simulink model "mymodel1"  (R2018a)
settings: Solver=VariableStepAuto  StartTime=0.0  StopTime=10.0  RelTol=1e-3
libraries: xbsIndex_r4 x12453, casper_library_misc x30, casper_library_delays x14, xps_library x2
(part 21 of 108)

== system mymodel1/pfb_fir_generic/pfb_fir_taps/bus_mult ==
  a : Inport
  b : Inport  Port=2
  a*b_bussify : Subsystem  AncestorBlock=casper_library_flow_control/bus_create  mask(bus_create){inputNum=96}
      mask prompts: inputNum "Number of inputs:"
      mask init:
      | bus_create_init(gcb,...
      |     'inputNum', inputNum);
  a_debus : Subsystem  AncestorBlock=casper_library_flow_control/bus_expand  mask(bus_expand){mode=divisions of arbitrary size, outputNum=1, outputWidth=[16 16 16 16 16 16 16 16 16 16 16 16 16 16 16 16 16 16 16 16 16 16 16 16 16 16 16 16 16 16 16 16 16 16 16 16 16 16 16 16 16 16 16 16 16 16 16 16 16 16 16 16 16 16 16 16 16 16 16 16 16 16 16 16 16 16 16 16 16 16 16 16 16 16 16 16 16 16 16 16 16 16 16 16 16 16 16 16 16 16 16 16 16 16 16 16], outputBinaryPt=[15 15 15 15 15 15 15 15 15 15 15 15 15 15 15 15 15 15 15 15 15 15 15 15 15 15 15 15 15 15 15 15 15 15 15 15 15 15 15 15 15 15 15 15 15 15 15 15 15 15 15 15 15 15 15 15 15 15 15 15 15 15 15 15 15 15 15 15 15 15 15 15 15 15 15 15 15 15 15 15 15 15 15 15 15 15 15 15 15 15 15 15 15 15 15 15], outputArithmeticType=[1 1 1 1 1 1 1 1 1 1 1 1 1 1 1 1 1 1 1 1 1 1 1 1 1 1 1 1 1 1 1 1 1 1 1 1 1 1 1 1 1 1 1 1 1 1 1 1 1 1 1 1 1 1 1 1 1 1 1 1 1 1 1 1 1 1 1 1 1 1 1 1 1 1 1 1 1 1 1 1 1 1 1 1 1 1 1 1 1 1 1 1 1 1 1 1], show_format=on, outputToWorkspace=off, variablePrefix=, outputToModelAsWell=on}
      mask prompts: outputNum "Number of outputs:"; outputWidth "Output width [msb ... lsb]:"; outputBinaryPt "Output binary point position [msb ... lsb]:"; outputArithmeticType "Output arithmetic type (ufix=0, fix=1, bool=2) [msb ... lsb]:"; show_format "Print format string?"; outputToWorkspace "Output to workspace?"; variablePrefix "Variable name prefix:"; outputToModelAsWell "Output to model as well?"
      mask help:
      | Expands a 'bus' made using a bus_create or Xilinx
      | concat block.
      | The input will be divided into the specified number
      | of outputs with the specified arithmetic types.
      | Divisions are made from most significant bit.
      mask init: same as mymodel1/bit_sel_xx0/bus_expand1
      settings: AttributesFormatString=96 outputs: f16.15,f16.15,f16.15,f16.15,f16.15,f16.15,f16.15,f16.15,f16.15,f16.15,f16.15,f16.15,f16.15,f16.15,f16.15,f16.15,f16.15,f16.15,f16.15,f16.15,f16.15,f16.15,f16.15,f16.15,f16.15,f16.15,f16.15,f16.15,f16.15,f16.15,f16.15,f16.15,f16.15,f16.15,f16.15,f16.15,f16.15,f16.15,f16.15,f16.15,f16.15,f16.15,f16.15,f16.15,f16.15,f16.15,f16.15,f16.15,f16.15,f16.15,f16.15,f16.15,f16.15,f16.15,f16.15,f16.15,f16.15,f16.15,f16.15,f16.15,f16.15,f16.15,f16.15,f16.15,f16.15,f16.15,f16.15,f16.15,f16.15,f16.15,f16.15,f16.15,f16.15,f16.15,f16.15,f16.15,f16.15,f16.15,f16.15,f16.15,f16.15,f16.15,f16.15,f16.15,f16.15,f16.15,f16.15,f16.15,f16.15,f16.15,f16.15,f16.15,f16.15,f16.15,f16.15,f16.15,
      mask TypeOptions mode: divisions of equal size | divisions of arbitrary size
      mask Callback mode: bus_expand_callback();
      mask Callback outputWidth: bus_expand_callback();
      mask Callback outputToWorkspace: bus_expand_callback();
  b_debus : Subsystem  AncestorBlock=casper_library_flow_control/bus_expand  mask(bus_expand){mode=divisions of arbitrary size, outputNum=1, outputWidth=[18 18 18 18 18 18 18 18 18 18 18 18 18 18 18 18 18 18 18 18 18 18 18 18 18 18 18 18 18 18 18 18 18 18 18 18 18 18 18 18 18 18 18 18 18 18 18 18 18 18 18 18 18 18 18 18 18 18 18 18 18 18 18 18 18 18 18 18 18 18 18 18 18 18 18 18 18 18 18 18 18 18 18 18 18 18 18 18 18 18 18 18 18 18 18 18], outputBinaryPt=[17 17 17 17 17 17 17 17 17 17 17 17 17 17 17 17 17 17 17 17 17 17 17 17 17 17 17 17 17 17 17 17 17 17 17 17 17 17 17 17 17 17 17 17 17 17 17 17 17 17 17 17 17 17 17 17 17 17 17 17 17 17 17 17 17 17 17 17 17 17 17 17 17 17 17 17 17 17 17 17 17 17 17 17 17 17 17 17 17 17 17 17 17 17 17 17], outputArithmeticType=[1 1 1 1 1 1 1 1 1 1 1 1 1 1 1 1 1 1 1 1 1 1 1 1 1 1 1 1 1 1 1 1 1 1 1 1 1 1 1 1 1 1 1 1 1 1 1 1 1 1 1 1 1 1 1 1 1 1 1 1 1 1 1 1 1 1 1 1 1 1 1 1 1 1 1 1 1 1 1 1 1 1 1 1 1 1 1 1 1 1 1 1 1 1 1 1], show_format=on, outputToWorkspace=off, variablePrefix=, outputToModelAsWell=on}
      mask prompts: outputNum "Number of outputs:"; outputWidth "Output width [msb ... lsb]:"; outputBinaryPt "Output binary point position [msb ... lsb]:"; outputArithmeticType "Output arithmetic type (ufix=0, fix=1, bool=2) [msb ... lsb]:"; show_format "Print format string?"; outputToWorkspace "Output to workspace?"; variablePrefix "Variable name prefix:"; outputToModelAsWell "Output to model as well?"
      mask help:
      | Expands a 'bus' made using a bus_create or Xilinx
      | concat block.
      | The input will be divided into the specified number
      | of outputs with the specified arithmetic types.
      | Divisions are made from most significant bit.
      mask init: same as mymodel1/bit_sel_xx0/bus_expand1
      settings: AttributesFormatString=96 outputs: f18.17,f18.17,f18.17,f18.17,f18.17,f18.17,f18.17,f18.17,f18.17,f18.17,f18.17,f18.17,f18.17,f18.17,f18.17,f18.17,f18.17,f18.17,f18.17,f18.17,f18.17,f18.17,f18.17,f18.17,f18.17,f18.17,f18.17,f18.17,f18.17,f18.17,f18.17,f18.17,f18.17,f18.17,f18.17,f18.17,f18.17,f18.17,f18.17,f18.17,f18.17,f18.17,f18.17,f18.17,f18.17,f18.17,f18.17,f18.17,f18.17,f18.17,f18.17,f18.17,f18.17,f18.17,f18.17,f18.17,f18.17,f18.17,f18.17,f18.17,f18.17,f18.17,f18.17,f18.17,f18.17,f18.17,f18.17,f18.17,f18.17,f18.17,f18.17,f18.17,f18.17,f18.17,f18.17,f18.17,f18.17,f18.17,f18.17,f18.17,f18.17,f18.17,f18.17,f18.17,f18.17,f18.17,f18.17,f18.17,f18.17,f18.17,f18.17,f18.17,f18.17,f18.17,f18.17,f18.17,
      mask TypeOptions mode: divisions of equal size | divisions of arbitrary size
      mask Callback mode: bus_expand_callback();
      mask Callback outputWidth: bus_expand_callback();
      mask Callback outputToWorkspace: bus_expand_callback();
  mult{1..96} (96 alike) : xbsIndex_r4/Mult  precision=User Defined  arith_type="Signed  (2's comp)"  n_bits=34  bin_pt=32  quantization=Truncate  overflow=Wrap  en=off  latency=mult_latency  use_behavioral_HDL=on  opt=Speed  use_embedded=off  optimum_pipeline=off  pipeline=on  dbl_ovrd=off  use_rpm=on  placement_style=Triangular  block_type=mult
  repa : Subsystem  AncestorBlock=casper_library_bus/bus_replicate  mask(bus_replicate){replication=1, csp_latency=0, misc=off, implementation=core}
      mask prompts: replication "replication factor"; csp_latency "latency"; misc "misc support"; implementation "delay implementation"
      mask help: Output bus formed by replicating input bus a number of times
      mask init:
      | bus_replicate_init(gcb, ...
      |     'replication', replication, ...
      |     'csp_latency', csp_latency, ...
      |     'implementation', implementation, ...
      |     'misc', misc);
      mask TypeOptions implementation: core | behavioral
  repb : Subsystem  AncestorBlock=casper_library_bus/bus_replicate  mask(bus_replicate){replication=1, csp_latency=0, misc=off, implementation=core}
      mask prompts: replication "replication factor"; csp_latency "latency"; misc "misc support"; implementation "delay implementation"
      mask help: Output bus formed by replicating input bus a number of times
      mask init:
      | bus_replicate_init(gcb, ...
      |     'replication', replication, ...
      |     'csp_latency', csp_latency, ...
      |     'implementation', implementation, ...
      |     'misc', misc);
      mask TypeOptions implementation: core | behavioral
  a*b : Outport
  wires:
  a/1 -> repa/1(in)
  b/1 -> repb/1(in)
  repa/1(out) -> a_debus/1(bus_in)
  repb/1(out) -> b_debus/1(bus_in)
  a_debus/1(msb_out96) -> mult1/1
  b_debus/1(msb_out96) -> mult1/2
  a_debus/2(out95) -> mult2/1
  b_debus/2(out95) -> mult2/2
  a_debus/3(out94) -> mult3/1
  b_debus/3(out94) -> mult3/2
  a_debus/4(out93) -> mult4/1
  b_debus/4(out93) -> mult4/2
  a_debus/5(out92) -> mult5/1
  b_debus/5(out92) -> mult5/2
  a_debus/6(out91) -> mult6/1
  b_debus/6(out91) -> mult6/2
  a_debus/7(out90) -> mult7/1
  b_debus/7(out90) -> mult7/2
  a_debus/8(out89) -> mult8/1
  b_debus/8(out89) -> mult8/2
  a_debus/9(out88) -> mult9/1
  b_debus/9(out88) -> mult9/2
  a_debus/10(out87) -> mult10/1
  b_debus/10(out87) -> mult10/2
  a_debus/11(out86) -> mult11/1
  b_debus/11(out86) -> mult11/2
  a_debus/12(out85) -> mult12/1
  b_debus/12(out85) -> mult12/2
  a_debus/13(out84) -> mult13/1
  b_debus/13(out84) -> mult13/2
  a_debus/14(out83) -> mult14/1
  b_debus/14(out83) -> mult14/2
  a_debus/15(out82) -> mult15/1
  b_debus/15(out82) -> mult15/2
  a_debus/16(out81) -> mult16/1
  b_debus/16(out81) -> mult16/2
  a_debus/17(out80) -> mult17/1
  b_debus/17(out80) -> mult17/2
  a_debus/18(out79) -> mult18/1
  b_debus/18(out79) -> mult18/2
  a_debus/19(out78) -> mult19/1
  b_debus/19(out78) -> mult19/2
  a_debus/20(out77) -> mult20/1
  b_debus/20(out77) -> mult20/2
  a_debus/21(out76) -> mult21/1
  b_debus/21(out76) -> mult21/2
  a_debus/22(out75) -> mult22/1
  b_debus/22(out75) -> mult22/2
  a_debus/23(out74) -> mult23/1
  b_debus/23(out74) -> mult23/2
  a_debus/24(out73) -> mult24/1
  b_debus/24(out73) -> mult24/2
  a_debus/25(out72) -> mult25/1
  b_debus/25(out72) -> mult25/2
  a_debus/26(out71) -> mult26/1
  b_debus/26(out71) -> mult26/2
  a_debus/27(out70) -> mult27/1
  b_debus/27(out70) -> mult27/2
  a_debus/28(out69) -> mult28/1
  b_debus/28(out69) -> mult28/2
  a_debus/29(out68) -> mult29/1
  b_debus/29(out68) -> mult29/2
  a_debus/30(out67) -> mult30/1
  b_debus/30(out67) -> mult30/2
  a_debus/31(out66) -> mult31/1
  b_debus/31(out66) -> mult31/2
  a_debus/32(out65) -> mult32/1
  b_debus/32(out65) -> mult32/2
  a_debus/33(out64) -> mult33/1
  b_debus/33(out64) -> mult33/2
  a_debus/34(out63) -> mult34/1
  b_debus/34(out63) -> mult34/2
  a_debus/35(out62) -> mult35/1
  b_debus/35(out62) -> mult35/2
  a_debus/36(out61) -> mult36/1
  b_debus/36(out61) -> mult36/2
  a_debus/37(out60) -> mult37/1
  b_debus/37(out60) -> mult37/2
  a_debus/38(out59) -> mult38/1
  b_debus/38(out59) -> mult38/2
  a_debus/39(out58) -> mult39/1
  b_debus/39(out58) -> mult39/2
  a_debus/40(out57) -> mult40/1
  b_debus/40(out57) -> mult40/2
  a_debus/41(out56) -> mult41/1
  b_debus/41(out56) -> mult41/2
  a_debus/42(out55) -> mult42/1
  b_debus/42(out55) -> mult42/2
  a_debus/43(out54) -> mult43/1
  b_debus/43(out54) -> mult43/2
  a_debus/44(out53) -> mult44/1
  b_debus/44(out53) -> mult44/2
  a_debus/45(out52) -> mult45/1
  b_debus/45(out52) -> mult45/2
  a_debus/46(out51) -> mult46/1
  b_debus/46(out51) -> mult46/2
  a_debus/47(out50) -> mult47/1
  b_debus/47(out50) -> mult47/2
  a_debus/48(out49) -> mult48/1
  b_debus/48(out49) -> mult48/2
  a_debus/49(out48) -> mult49/1
  b_debus/49(out48) -> mult49/2
  a_debus/50(out47) -> mult50/1
  b_debus/50(out47) -> mult50/2
  a_debus/51(out46) -> mult51/1
  b_debus/51(out46) -> mult51/2
  a_debus/52(out45) -> mult52/1
  b_debus/52(out45) -> mult52/2
  a_debus/53(out44) -> mult53/1
  b_debus/53(out44) -> mult53/2
  a_debus/54(out43) -> mult54/1
  b_debus/54(out43) -> mult54/2
  a_debus/55(out42) -> mult55/1
  b_debus/55(out42) -> mult55/2
  a_debus/56(out41) -> mult56/1
  b_debus/56(out41) -> mult56/2
  a_debus/57(out40) -> mult57/1
  b_debus/57(out40) -> mult57/2
  a_debus/58(out39) -> mult58/1
  b_debus/58(out39) -> mult58/2
  a_debus/59(out38) -> mult59/1
  b_debus/59(out38) -> mult59/2
  a_debus/60(out37) -> mult60/1
  b_debus/60(out37) -> mult60/2
  a_debus/61(out36) -> mult61/1
  b_debus/61(out36) -> mult61/2
  a_debus/62(out35) -> mult62/1
  b_debus/62(out35) -> mult62/2
  a_debus/63(out34) -> mult63/1
  b_debus/63(out34) -> mult63/2
  a_debus/64(out33) -> mult64/1
  b_debus/64(out33) -> mult64/2
  a_debus/65(out32) -> mult65/1
  b_debus/65(out32) -> mult65/2
  a_debus/66(out31) -> mult66/1
  b_debus/66(out31) -> mult66/2
  a_debus/67(out30) -> mult67/1
  b_debus/67(out30) -> mult67/2
  a_debus/68(out29) -> mult68/1
  b_debus/68(out29) -> mult68/2
  a_debus/69(out28) -> mult69/1
  b_debus/69(out28) -> mult69/2
  a_debus/70(out27) -> mult70/1
  b_debus/70(out27) -> mult70/2
  a_debus/71(out26) -> mult71/1
  b_debus/71(out26) -> mult71/2
  a_debus/72(out25) -> mult72/1
  b_debus/72(out25) -> mult72/2
  a_debus/73(out24) -> mult73/1
  b_debus/73(out24) -> mult73/2
  a_debus/74(out23) -> mult74/1
  b_debus/74(out23) -> mult74/2
  a_debus/75(out22) -> mult75/1
  b_debus/75(out22) -> mult75/2
  a_debus/76(out21) -> mult76/1
  b_debus/76(out21) -> mult76/2
  a_debus/77(out20) -> mult77/1
  b_debus/77(out20) -> mult77/2
  a_debus/78(out19) -> mult78/1
  b_debus/78(out19) -> mult78/2
  a_debus/79(out18) -> mult79/1
  b_debus/79(out18) -> mult79/2
  a_debus/80(out17) -> mult80/1
  b_debus/80(out17) -> mult80/2
  a_debus/81(out16) -> mult81/1
  b_debus/81(out16) -> mult81/2
  a_debus/82(out15) -> mult82/1
  b_debus/82(out15) -> mult82/2
  a_debus/83(out14) -> mult83/1
  b_debus/83(out14) -> mult83/2
  a_debus/84(out13) -> mult84/1
  b_debus/84(out13) -> mult84/2
  a_debus/85(out12) -> mult85/1
  b_debus/85(out12) -> mult85/2
  a_debus/86(out11) -> mult86/1
  b_debus/86(out11) -> mult86/2
  a_debus/87(out10) -> mult87/1
  b_debus/87(out10) -> mult87/2
  a_debus/88(out9) -> mult88/1
  b_debus/88(out9) -> mult88/2
  a_debus/89(out8) -> mult89/1
  b_debus/89(out8) -> mult89/2
  a_debus/90(out7) -> mult90/1
  b_debus/90(out7) -> mult90/2
  a_debus/91(out6) -> mult91/1
  b_debus/91(out6) -> mult91/2
  a_debus/92(out5) -> mult92/1
  b_debus/92(out5) -> mult92/2
  a_debus/93(out4) -> mult93/1
  b_debus/93(out4) -> mult93/2
  a_debus/94(out3) -> mult94/1
  b_debus/94(out3) -> mult94/2
  a_debus/95(out2) -> mult95/1
  b_debus/95(out2) -> mult95/2
  a_debus/96(lsb_out1) -> mult96/1
  b_debus/96(lsb_out1) -> mult96/2
  mult1/1 -> a*b_bussify/1(in1)
  mult2/1 -> a*b_bussify/2(in2)
  mult3/1 -> a*b_bussify/3(in3)
  mult4/1 -> a*b_bussify/4(in4)
  mult5/1 -> a*b_bussify/5(in5)
  mult6/1 -> a*b_bussify/6(in6)
  mult7/1 -> a*b_bussify/7(in7)
  mult8/1 -> a*b_bussify/8(in8)
  mult9/1 -> a*b_bussify/9(in9)
  mult10/1 -> a*b_bussify/10(in10)
  mult11/1 -> a*b_bussify/11(in11)
  mult12/1 -> a*b_bussify/12(in12)
  mult13/1 -> a*b_bussify/13(in13)
  mult14/1 -> a*b_bussify/14(in14)
  mult15/1 -> a*b_bussify/15(in15)
  mult16/1 -> a*b_bussify/16(in16)
  mult17/1 -> a*b_bussify/17(in17)
  mult18/1 -> a*b_bussify/18(in18)
  mult19/1 -> a*b_bussify/19(in19)
  mult20/1 -> a*b_bussify/20(in20)
  mult21/1 -> a*b_bussify/21(in21)
  mult22/1 -> a*b_bussify/22(in22)
  mult23/1 -> a*b_bussify/23(in23)
  mult24/1 -> a*b_bussify/24(in24)
  mult25/1 -> a*b_bussify/25(in25)
  mult26/1 -> a*b_bussify/26(in26)
  mult27/1 -> a*b_bussify/27(in27)
  mult28/1 -> a*b_bussify/28(in28)
  mult29/1 -> a*b_bussify/29(in29)
  mult30/1 -> a*b_bussify/30(in30)
  mult31/1 -> a*b_bussify/31(in31)
  mult32/1 -> a*b_bussify/32(in32)
  mult33/1 -> a*b_bussify/33(in33)
  mult34/1 -> a*b_bussify/34(in34)
  mult35/1 -> a*b_bussify/35(in35)
  mult36/1 -> a*b_bussify/36(in36)
  mult37/1 -> a*b_bussify/37(in37)
  mult38/1 -> a*b_bussify/38(in38)
  mult39/1 -> a*b_bussify/39(in39)
  mult40/1 -> a*b_bussify/40(in40)
  mult41/1 -> a*b_bussify/41(in41)
  mult42/1 -> a*b_bussify/42(in42)
  mult43/1 -> a*b_bussify/43(in43)
  mult44/1 -> a*b_bussify/44(in44)
  mult45/1 -> a*b_bussify/45(in45)
  mult46/1 -> a*b_bussify/46(in46)
  mult47/1 -> a*b_bussify/47(in47)
  mult48/1 -> a*b_bussify/48(in48)
  mult49/1 -> a*b_bussify/49(in49)
  mult50/1 -> a*b_bussify/50(in50)
  mult51/1 -> a*b_bussify/51(in51)
  mult52/1 -> a*b_bussify/52(in52)
  mult53/1 -> a*b_bussify/53(in53)
  mult54/1 -> a*b_bussify/54(in54)
  mult55/1 -> a*b_bussify/55(in55)
  mult56/1 -> a*b_bussify/56(in56)
  mult57/1 -> a*b_bussify/57(in57)
  mult58/1 -> a*b_bussify/58(in58)
  mult59/1 -> a*b_bussify/59(in59)
  mult60/1 -> a*b_bussify/60(in60)
  mult61/1 -> a*b_bussify/61(in61)
  mult62/1 -> a*b_bussify/62(in62)
  mult63/1 -> a*b_bussify/63(in63)
  mult64/1 -> a*b_bussify/64(in64)
  mult65/1 -> a*b_bussify/65(in65)
  mult66/1 -> a*b_bussify/66(in66)
  mult67/1 -> a*b_bussify/67(in67)
  mult68/1 -> a*b_bussify/68(in68)
  mult69/1 -> a*b_bussify/69(in69)
  mult70/1 -> a*b_bussify/70(in70)
  mult71/1 -> a*b_bussify/71(in71)
  mult72/1 -> a*b_bussify/72(in72)
  mult73/1 -> a*b_bussify/73(in73)
  mult74/1 -> a*b_bussify/74(in74)
  mult75/1 -> a*b_bussify/75(in75)
  mult76/1 -> a*b_bussify/76(in76)
  mult77/1 -> a*b_bussify/77(in77)
  mult78/1 -> a*b_bussify/78(in78)
  mult79/1 -> a*b_bussify/79(in79)
  mult80/1 -> a*b_bussify/80(in80)
  mult81/1 -> a*b_bussify/81(in81)
  mult82/1 -> a*b_bussify/82(in82)
  mult83/1 -> a*b_bussify/83(in83)
  mult84/1 -> a*b_bussify/84(in84)
  mult85/1 -> a*b_bussify/85(in85)
  mult86/1 -> a*b_bussify/86(in86)
  mult87/1 -> a*b_bussify/87(in87)
  mult88/1 -> a*b_bussify/88(in88)
  mult89/1 -> a*b_bussify/89(in89)
  mult90/1 -> a*b_bussify/90(in90)
  mult91/1 -> a*b_bussify/91(in91)
  mult92/1 -> a*b_bussify/92(in92)
  mult93/1 -> a*b_bussify/93(in93)
  mult94/1 -> a*b_bussify/94(in94)
  mult95/1 -> a*b_bussify/95(in95)
  mult96/1 -> a*b_bussify/96(in96)
  a*b_bussify/1(bus_out) -> a*b/1

== system mymodel1/pfb_fir_generic/pfb_fir_taps/tap_delays ==
  addra : Inport
  dina : Inport  Port=2
  wea : Inport  Port=3
  addrb : Inport  Port=4
  dinb : Inport  Port=5
  web : Inport  Port=6
  A_bussify0 : Subsystem  AncestorBlock=casper_library_flow_control/bus_create  mask(bus_create){inputNum=40}
      mask prompts: inputNum "Number of inputs:"
      mask init:
      | bus_create_init(gcb,...
      |     'inputNum', inputNum);
  B_bussify0 : Subsystem  AncestorBlock=casper_library_flow_control/bus_create  mask(bus_create){inputNum=40}
      mask prompts: inputNum "Number of inputs:"
      mask init:
      | bus_create_init(gcb,...
      |     'inputNum', inputNum);
  alsbs_slice : xbsIndex_r4/Slice  nbits=10  boolean_output=off  mode=Lower Bit Location + Width  bit1=0  base1=LSB of Input  bit0=0  base0=LSB of Input  dbl_ovrd=off  block_type=slice
  blsbs_slice : xbsIndex_r4/Slice  nbits=10  boolean_output=off  mode=Lower Bit Location + Width  bit1=0  base1=LSB of Input  bit0=0  base0=LSB of Input  dbl_ovrd=off  block_type=slice
  bram0_{0..39} (40 alike) : xbsIndex_r4/Dual Port RAM  depth=1024  initVector=getfield(get_param(gcb, 'UserData'), 'initVector')  distributed_mem=Block RAM  init_a=0  init_b=0  rst_a=off  rst_b=off  en_a=off  en_b=off  latency=2  write_mode_A=Read Before Write  write_mode_B=Read Before Write  optimize=Area  dbl_ovrd=off  block_type=dpram
  ddina0 : xbsIndex_r4/Delay  rst=off  infoeditControl=Selection of Reset will increase slice count due to use of real FFs and instead of SRLs  en=off  latency=0  reg_retiming=on  dbl_ovrd=off  block_type=delay
  ddinb0 : xbsIndex_r4/Delay  rst=off  infoeditControl=Selection of Reset will increase slice count due to use of real FFs and instead of SRLs  en=off  latency=1  reg_retiming=off  dbl_ovrd=off  block_type=delay
  debus_addra0 : Subsystem  AncestorBlock=casper_library_flow_control/bus_expand  mask(bus_expand){mode=divisions of equal size, outputNum=40, outputWidth=[10 10 10 10 10 10 10 10 10 10 10 10 10 10 10 10 10 10 10 10 10 10 10 10 10 10 10 10 10 10 10 10 10 10 10 10 10 10 10 10], outputBinaryPt=[0 0 0 0 0 0 0 0 0 0 0 0 0 0 0 0 0 0 0 0 0 0 0 0 0 0 0 0 0 0 0 0 0 0 0 0 0 0 0 0], outputArithmeticType=[0 0 0 0 0 0 0 0 0 0 0 0 0 0 0 0 0 0 0 0 0 0 0 0 0 0 0 0 0 0 0 0 0 0 0 0 0 0 0 0], show_format=on, outputToWorkspace=off, variablePrefix=, outputToModelAsWell=on}
      mask prompts: outputNum "Number of outputs:"; outputWidth "Output width:"; outputBinaryPt "Output binary point position:"; outputArithmeticType "Output arithmetic type (ufix=0, fix=1, bool=2):"; show_format "Print format string?"; outputToWorkspace "Output to workspace?"; variablePrefix "Variable name prefix:"; outputToModelAsWell "Output to model as well?"
      mask help:
      | Expands a 'bus' made using a bus_create or Xilinx
      | concat block.
      | The input will be divided into the specified number
      | of outputs with the specified arithmetic types.
      | Divisions are made from most significant bit.
      mask init: same as mymodel1/bit_sel_xx0/bus_expand1
      settings: AttributesFormatString=40 outputs: uf10.0,uf10.0,uf10.0,uf10.0,uf10.0,uf10.0,uf10.0,uf10.0,uf10.0,uf10.0,uf10.0,uf10.0,uf10.0,uf10.0,uf10.0,uf10.0,uf10.0,uf10.0,uf10.0,uf10.0,uf10.0,uf10.0,uf10.0,uf10.0,uf10.0,uf10.0,uf10.0,uf10.0,uf10.0,uf10.0,uf10.0,uf10.0,uf10.0,uf10.0,uf10.0,uf10.0,uf10.0,uf10.0,uf10.0,uf10.0,
      mask TypeOptions mode: divisions of equal size | divisions of arbitrary size
      mask Callback mode: bus_expand_callback();
      mask Callback outputWidth: bus_expand_callback();
      mask Callback outputToWorkspace: bus_expand_callback();
  debus_addrb0 : Subsystem  AncestorBlock=casper_library_flow_control/bus_expand  mask(bus_expand){mode=divisions of equal size, outputNum=40, outputWidth=[10 10 10 10 10 10 10 10 10 10 10 10 10 10 10 10 10 10 10 10 10 10 10 10 10 10 10 10 10 10 10 10 10 10 10 10 10 10 10 10], outputBinaryPt=[0 0 0 0 0 0 0 0 0 0 0 0 0 0 0 0 0 0 0 0 0 0 0 0 0 0 0 0 0 0 0 0 0 0 0 0 0 0 0 0], outputArithmeticType=[0 0 0 0 0 0 0 0 0 0 0 0 0 0 0 0 0 0 0 0 0 0 0 0 0 0 0 0 0 0 0 0 0 0 0 0 0 0 0 0], show_format=on, outputToWorkspace=off, variablePrefix=, outputToModelAsWell=on}
      mask prompts: outputNum "Number of outputs:"; outputWidth "Output width:"; outputBinaryPt "Output binary point position:"; outputArithmeticType "Output arithmetic type (ufix=0, fix=1, bool=2):"; show_format "Print format string?"; outputToWorkspace "Output to workspace?"; variablePrefix "Variable name prefix:"; outputToModelAsWell "Output to model as well?"
      mask help:
      | Expands a 'bus' made using a bus_create or Xilinx
      | concat block.
      | The input will be divided into the specified number
      | of outputs with the specified arithmetic types.
      | Divisions are made from most significant bit.
      mask init: same as mymodel1/bit_sel_xx0/bus_expand1
      settings: AttributesFormatString=40 outputs: uf10.0,uf10.0,uf10.0,uf10.0,uf10.0,uf10.0,uf10.0,uf10.0,uf10.0,uf10.0,uf10.0,uf10.0,uf10.0,uf10.0,uf10.0,uf10.0,uf10.0,uf10.0,uf10.0,uf10.0,uf10.0,uf10.0,uf10.0,uf10.0,uf10.0,uf10.0,uf10.0,uf10.0,uf10.0,uf10.0,uf10.0,uf10.0,uf10.0,uf10.0,uf10.0,uf10.0,uf10.0,uf10.0,uf10.0,uf10.0,
      mask TypeOptions mode: divisions of equal size | divisions of arbitrary size
      mask Callback mode: bus_expand_callback();
      mask Callback outputWidth: bus_expand_callback();
      mask Callback outputToWorkspace: bus_expand_callback();
  debus_dina0 : Subsystem  AncestorBlock=casper_library_flow_control/bus_expand  mask(bus_expand){mode=divisions of arbitrary size, outputNum=1, outputWidth=[4 36 36 36 36 36 36 36 36 36 36 36 36 36 36 36 36 36 36 36 36 36 36 36 36 36 36 36 36 36 36 36 36 36 36 36 36 36 36 36], outputBinaryPt=[0 0 0 0 0 0 0 0 0 0 0 0 0 0 0 0 0 0 0 0 0 0 0 0 0 0 0 0 0 0 0 0 0 0 0 0 0 0 0 0], outputArithmeticType=[0 0 0 0 0 0 0 0 0 0 0 0 0 0 0 0 0 0 0 0 0 0 0 0 0 0 0 0 0 0 0 0 0 0 0 0 0 0 0 0], show_format=on, outputToWorkspace=off, variablePrefix=, outputToModelAsWell=on}
      mask prompts: outputNum "Number of outputs:"; outputWidth "Output width [msb ... lsb]:"; outputBinaryPt "Output binary point position [msb ... lsb]:"; outputArithmeticType "Output arithmetic type (ufix=0, fix=1, bool=2) [msb ... lsb]:"; show_format "Print format string?"; outputToWorkspace "Output to workspace?"; variablePrefix "Variable name prefix:"; outputToModelAsWell "Output to model as well?"
      mask help:
      | Expands a 'bus' made using a bus_create or Xilinx
      | concat block.
      | The input will be divided into the specified number
      | of outputs with the specified arithmetic types.
      | Divisions are made from most significant bit.
      mask init: same as mymodel1/bit_sel_xx0/bus_expand1
      settings: AttributesFormatString=40 outputs: uf4.0,uf36.0,uf36.0,uf36.0,uf36.0,uf36.0,uf36.0,uf36.0,uf36.0,uf36.0,uf36.0,uf36.0,uf36.0,uf36.0,uf36.0,uf36.0,uf36.0,uf36.0,uf36.0,uf36.0,uf36.0,uf36.0,uf36.0,uf36.0,uf36.0,uf36.0,uf36.0,uf36.0,uf36.0,uf36.0,uf36.0,uf36.0,uf36.0,uf36.0,uf36.0,uf36.0,uf36.0,uf36.0,uf36.0,uf36.0,
      mask TypeOptions mode: divisions of equal size | divisions of arbitrary size
      mask Callback mode: bus_expand_callback();
      mask Callback outputWidth: bus_expand_callback();
      mask Callback outputToWorkspace: bus_expand_callback();
  debus_dinb0 : Subsystem  AncestorBlock=casper_library_flow_control/bus_expand  mask(bus_expand){mode=divisions of arbitrary size, outputNum=1, outputWidth=[4 36 36 36 36 36 36 36 36 36 36 36 36 36 36 36 36 36 36 36 36 36 36 36 36 36 36 36 36 36 36 36 36 36 36 36 36 36 36 36], outputBinaryPt=[0 0 0 0 0 0 0 0 0 0 0 0 0 0 0 0 0 0 0 0 0 0 0 0 0 0 0 0 0 0 0 0 0 0 0 0 0 0 0 0], outputArithmeticType=[0 0 0 0 0 0 0 0 0 0 0 0 0 0 0 0 0 0 0 0 0 0 0 0 0 0 0 0 0 0 0 0 0 0 0 0 0 0 0 0], show_format=on, outputToWorkspace=off, variablePrefix=, outputToModelAsWell=on}
      mask prompts: outputNum "Number of outputs:"; outputWidth "Output width [msb ... lsb]:"; outputBinaryPt "Output binary point position [msb ... lsb]:"; outputArithmeticType "Output arithmetic type (ufix=0, fix=1, bool=2) [msb ... lsb]:"; show_format "Print format string?"; outputToWorkspace "Output to workspace?"; variablePrefix "Variable name prefix:"; outputToModelAsWell "Output to model as well?"
      mask help:
      | Expands a 'bus' made using a bus_create or Xilinx
      | concat block.
      | The input will be divided into the specified number
      | of outputs with the specified arithmetic types.
      | Divisions are made from most significant bit.
      mask init: same as mymodel1/bit_sel_xx0/bus_expand1
      settings: AttributesFormatString=40 outputs: uf4.0,uf36.0,uf36.0,uf36.0,uf36.0,uf36.0,uf36.0,uf36.0,uf36.0,uf36.0,uf36.0,uf36.0,uf36.0,uf36.0,uf36.0,uf36.0,uf36.0,uf36.0,uf36.0,uf36.0,uf36.0,uf36.0,uf36.0,uf36.0,uf36.0,uf36.0,uf36.0,uf36.0,uf36.0,uf36.0,uf36.0,uf36.0,uf36.0,uf36.0,uf36.0,uf36.0,uf36.0,uf36.0,uf36.0,uf36.0,
      mask TypeOptions mode: divisions of equal size | divisions of arbitrary size
      mask Callback mode: bus_expand_callback();
      mask Callback outputWidth: bus_expand_callback();
      mask Callback outputToWorkspace: bus_expand_callback();
  debus_wea0 : Subsystem  AncestorBlock=casper_library_flow_control/bus_expand  mask(bus_expand){mode=divisions of equal size, outputNum=40, outputWidth=[1 1 1 1 1 1 1 1 1 1 1 1 1 1 1 1 1 1 1 1 1 1 1 1 1 1 1 1 1 1 1 1 1 1 1 1 1 1 1 1], outputBinaryPt=[0 0 0 0 0 0 0 0 0 0 0 0 0 0 0 0 0 0 0 0 0 0 0 0 0 0 0 0 0 0 0 0 0 0 0 0 0 0 0 0], outputArithmeticType=[2 2 2 2 2 2 2 2 2 2 2 2 2 2 2 2 2 2 2 2 2 2 2 2 2 2 2 2 2 2 2 2 2 2 2 2 2 2 2 2], show_format=on, outputToWorkspace=off, variablePrefix=, outputToModelAsWell=on}
      mask prompts: outputNum "Number of outputs:"; outputWidth "Output width:"; outputBinaryPt "Output binary point position:"; outputArithmeticType "Output arithmetic type (ufix=0, fix=1, bool=2):"; show_format "Print format string?"; outputToWorkspace "Output to workspace?"; variablePrefix "Variable name prefix:"; outputToModelAsWell "Output to model as well?"
      mask help:
      | Expands a 'bus' made using a bus_create or Xilinx
      | concat block.
      | The input will be divided into the specified number
      | of outputs with the specified arithmetic types.
      | Divisions are made from most significant bit.
      mask init: same as mymodel1/bit_sel_xx0/bus_expand1
      settings: AttributesFormatString=40 outputs: b,b,b,b,b,b,b,b,b,b,b,b,b,b,b,b,b,b,b,b,b,b,b,b,b,b,b,b,b,b,b,b,b,b,b,b,b,b,b,b,
      mask TypeOptions mode: divisions of equal size | divisions of arbitrary size
      mask Callback mode: bus_expand_callback();
      mask Callback outputWidth: bus_expand_callback();
      mask Callback outputToWorkspace: bus_expand_callback();
  debus_web0 : Subsystem  AncestorBlock=casper_library_flow_control/bus_expand  mask(bus_expand){mode=divisions of equal size, outputNum=40, outputWidth=[1 1 1 1 1 1 1 1 1 1 1 1 1 1 1 1 1 1 1 1 1 1 1 1 1 1 1 1 1 1 1 1 1 1 1 1 1 1 1 1], outputBinaryPt=[0 0 0 0 0 0 0 0 0 0 0 0 0 0 0 0 0 0 0 0 0 0 0 0 0 0 0 0 0 0 0 0 0 0 0 0 0 0 0 0], outputArithmeticType=[2 2 2 2 2 2 2 2 2 2 2 2 2 2 2 2 2 2 2 2 2 2 2 2 2 2 2 2 2 2 2 2 2 2 2 2 2 2 2 2], show_format=on, outputToWorkspace=off, variablePrefix=, outputToModelAsWell=on}
      mask prompts: outputNum "Number of outputs:"; outputWidth "Output width:"; outputBinaryPt "Output binary point position:"; outputArithmeticType "Output arithmetic type (ufix=0, fix=1, bool=2):"; show_format "Print format string?"; outputToWorkspace "Output to workspace?"; variablePrefix "Variable name prefix:"; outputToModelAsWell "Output to model as well?"
      mask help:
      | Expands a 'bus' made using a bus_create or Xilinx
      | concat block.
      | The input will be divided into the specified number
      | of outputs with the specified arithmetic types.
      | Divisions are made from most significant bit.
      mask init: same as mymodel1/bit_sel_xx0/bus_expand1
      settings: AttributesFormatString=40 outputs: b,b,b,b,b,b,b,b,b,b,b,b,b,b,b,b,b,b,b,b,b,b,b,b,b,b,b,b,b,b,b,b,b,b,b,b,b,b,b,b,
      mask TypeOptions mode: divisions of equal size | divisions of arbitrary size
      mask Callback mode: bus_expand_callback();
      mask Callback outputWidth: bus_expand_callback();
      mask Callback outputToWorkspace: bus_expand_callback();
  rep_addra0 : Subsystem  AncestorBlock=casper_library_bus/bus_replicate  mask(bus_replicate){replication=40, csp_latency=1, misc=off, implementation=core}
      mask prompts: replication "replication factor"; csp_latency "latency"; misc "misc support"; implementation "delay implementation"
      mask help: Output bus formed by replicating input bus a number of times
      mask init:
      | bus_replicate_init(gcb, ...
      |     'replication', replication, ...
      |     'csp_latency', csp_latency, ...
      |     'implementation', implementation, ...
      |     'misc', misc);
      mask TypeOptions implementation: core | behavioral
  rep_addrb0 : Subsystem  AncestorBlock=casper_library_bus/bus_replicate  mask(bus_replicate){replication=40, csp_latency=1, misc=off, implementation=core}
      mask prompts: replication "replication factor"; csp_latency "latency"; misc "misc support"; implementation "delay implementation"
      mask help: Output bus formed by replicating input bus a number of times
      mask init:
      | bus_replicate_init(gcb, ...
      |     'replication', replication, ...
      |     'csp_latency', csp_latency, ...
      |     'implementation', implementation, ...
      |     'misc', misc);
      mask TypeOptions implementation: core | behavioral
  rep_wea0 : Subsystem  AncestorBlock=casper_library_bus/bus_replicate  mask(bus_replicate){replication=40, csp_latency=0, misc=off, implementation=behavioral}
      mask prompts: replication "replication factor"; csp_latency "latency"; misc "misc support"; implementation "delay implementation"
      mask help: Output bus formed by replicating input bus a number of times
      mask init:
      | bus_replicate_init(gcb, ...
      |     'replication', replication, ...
      |     'csp_latency', csp_latency, ...
      |     'implementation', implementation, ...
      |     'misc', misc);
      mask TypeOptions implementation: core | behavioral
  rep_web0 : Subsystem  AncestorBlock=casper_library_bus/bus_replicate  mask(bus_replicate){replication=40, csp_latency=1, misc=off, implementation=core}
      mask prompts: replication "replication factor"; csp_latency "latency"; misc "misc support"; implementation "delay implementation"
      mask help: Output bus formed by replicating input bus a number of times
      mask init:
      | bus_replicate_init(gcb, ...
      |     'replication', replication, ...
      |     'csp_latency', csp_latency, ...
      |     'implementation', implementation, ...
      |     'misc', misc);
      mask TypeOptions implementation: core | behavioral
  A : Outport
  B : Outport  Port=2
  wires:
  addrb/1 -> blsbs_slice/1
  addra/1 -> alsbs_slice/1
  blsbs_slice/1 -> rep_addrb0/1(in)
  alsbs_slice/1 -> rep_addra0/1(in)
  dina/1 -> ddina0/1
  wea/1 -> rep_wea0/1(in)
  dinb/1 -> ddinb0/1
  web/1 -> rep_web0/1(in)
  rep_addrb0/1(out) -> debus_addrb0/1(bus_in)
  rep_addra0/1(out) -> debus_addra0/1(bus_in)
  ddina0/1 -> debus_dina0/1(bus_in)
  rep_wea0/1(out) -> debus_wea0/1(bus_in)
  ddinb0/1 -> debus_dinb0/1(bus_in)
  rep_web0/1(out) -> debus_web0/1(bus_in)
  debus_addra0/1(msb_out40) -> bram0_0/1
  debus_dina0/1(msb_out40) -> bram0_0/2
  debus_wea0/1(msb_out40) -> bram0_0/3
  debus_addrb0/1(msb_out40) -> bram0_0/4
  debus_dinb0/1(msb_out40) -> bram0_0/5
  debus_web0/1(msb_out40) -> bram0_0/6
  debus_addra0/2(out39) -> bram0_1/1
  debus_dina0/2(out39) -> bram0_1/2
  debus_wea0/2(out39) -> bram0_1/3
  debus_addrb0/2(out39) -> bram0_1/4
  debus_dinb0/2(out39) -> bram0_1/5
  debus_web0/2(out39) -> bram0_1/6
  debus_addra0/3(out38) -> bram0_2/1
  debus_dina0/3(out38) -> bram0_2/2
  debus_wea0/3(out38) -> bram0_2/3
  debus_addrb0/3(out38) -> bram0_2/4
  debus_dinb0/3(out38) -> bram0_2/5
  debus_web0/3(out38) -> bram0_2/6
  debus_addra0/4(out37) -> bram0_3/1
  debus_dina0/4(out37) -> bram0_3/2
  debus_wea0/4(out37) -> bram0_3/3
  debus_addrb0/4(out37) -> bram0_3/4
  debus_dinb0/4(out37) -> bram0_3/5
  debus_web0/4(out37) -> bram0_3/6
  debus_addra0/5(out36) -> bram0_4/1
  debus_dina0/5(out36) -> bram0_4/2
  debus_wea0/5(out36) -> bram0_4/3
  debus_addrb0/5(out36) -> bram0_4/4
  debus_dinb0/5(out36) -> bram0_4/5
  debus_web0/5(out36) -> bram0_4/6
  debus_addra0/6(out35) -> bram0_5/1
  debus_dina0/6(out35) -> bram0_5/2
  debus_wea0/6(out35) -> bram0_5/3
  debus_addrb0/6(out35) -> bram0_5/4
  debus_dinb0/6(out35) -> bram0_5/5
  debus_web0/6(out35) -> bram0_5/6
  debus_addra0/7(out34) -> bram0_6/1
  debus_dina0/7(out34) -> bram0_6/2
  debus_wea0/7(out34) -> bram0_6/3
  debus_addrb0/7(out34) -> bram0_6/4
  debus_dinb0/7(out34) -> bram0_6/5
  debus_web0/7(out34) -> bram0_6/6
  debus_addra0/8(out33) -> bram0_7/1
  debus_dina0/8(out33) -> bram0_7/2
  debus_wea0/8(out33) -> bram0_7/3
  debus_addrb0/8(out33) -> bram0_7/4
  debus_dinb0/8(out33) -> bram0_7/5
  debus_web0/8(out33) -> bram0_7/6
  debus_addra0/9(out32) -> bram0_8/1
  debus_dina0/9(out32) -> bram0_8/2
  debus_wea0/9(out32) -> bram0_8/3
  debus_addrb0/9(out32) -> bram0_8/4
  debus_dinb0/9(out32) -> bram0_8/5
  debus_web0/9(out32) -> bram0_8/6
  debus_addra0/10(out31) -> bram0_9/1
  debus_dina0/10(out31) -> bram0_9/2
  debus_wea0/10(out31) -> bram0_9/3
  debus_addrb0/10(out31) -> bram0_9/4
  debus_dinb0/10(out31) -> bram0_9/5
  debus_web0/10(out31) -> bram0_9/6
  debus_addra0/11(out30) -> bram0_10/1
  debus_dina0/11(out30) -> bram0_10/2
  debus_wea0/11(out30) -> bram0_10/3
  debus_addrb0/11(out30) -> bram0_10/4
  debus_dinb0/11(out30) -> bram0_10/5
  debus_web0/11(out30) -> bram0_10/6
  debus_addra0/12(out29) -> bram0_11/1
  debus_dina0/12(out29) -> bram0_11/2
  debus_wea0/12(out29) -> bram0_11/3
  debus_addrb0/12(out29) -> bram0_11/4
  debus_dinb0/12(out29) -> bram0_11/5
  debus_web0/12(out29) -> bram0_11/6
  debus_addra0/13(out28) -> bram0_12/1
  debus_dina0/13(out28) -> bram0_12/2
  debus_wea0/13(out28) -> bram0_12/3
  debus_addrb0/13(out28) -> bram0_12/4
  debus_dinb0/13(out28) -> bram0_12/5
  debus_web0/13(out28) -> bram0_12/6
  debus_addra0/14(out27) -> bram0_13/1
  debus_dina0/14(out27) -> bram0_13/2
  debus_wea0/14(out27) -> bram0_13/3
  debus_addrb0/14(out27) -> bram0_13/4
  debus_dinb0/14(out27) -> bram0_13/5
  debus_web0/14(out27) -> bram0_13/6
  debus_addra0/15(out26) -> bram0_14/1
  debus_dina0/15(out26) -> bram0_14/2
  debus_wea0/15(out26) -> bram0_14/3
  debus_addrb0/15(out26) -> bram0_14/4
  debus_dinb0/15(out26) -> bram0_14/5
  debus_web0/15(out26) -> bram0_14/6
  debus_addra0/16(out25) -> bram0_15/1
  debus_dina0/16(out25) -> bram0_15/2
  debus_wea0/16(out25) -> bram0_15/3
  debus_addrb0/16(out25) -> bram0_15/4
  debus_dinb0/16(out25) -> bram0_15/5
  debus_web0/16(out25) -> bram0_15/6
  debus_addra0/17(out24) -> bram0_16/1
  debus_dina0/17(out24) -> bram0_16/2
  debus_wea0/17(out24) -> bram0_16/3
  debus_addrb0/17(out24) -> bram0_16/4
  debus_dinb0/17(out24) -> bram0_16/5
  debus_web0/17(out24) -> bram0_16/6
  debus_addra0/18(out23) -> bram0_17/1
  debus_dina0/18(out23) -> bram0_17/2
  debus_wea0/18(out23) -> bram0_17/3
  debus_addrb0/18(out23) -> bram0_17/4
  debus_dinb0/18(out23) -> bram0_17/5
  debus_web0/18(out23) -> bram0_17/6
  debus_addra0/19(out22) -> bram0_18/1
  debus_dina0/19(out22) -> bram0_18/2
  debus_wea0/19(out22) -> bram0_18/3
  debus_addrb0/19(out22) -> bram0_18/4
  debus_dinb0/19(out22) -> bram0_18/5
  debus_web0/19(out22) -> bram0_18/6
  debus_addra0/20(out21) -> bram0_19/1
  debus_dina0/20(out21) -> bram0_19/2
  debus_wea0/20(out21) -> bram0_19/3
  debus_addrb0/20(out21) -> bram0_19/4
  debus_dinb0/20(out21) -> bram0_19/5
  debus_web0/20(out21) -> bram0_19/6
  debus_addra0/21(out20) -> bram0_20/1
  debus_dina0/21(out20) -> bram0_20/2
  debus_wea0/21(out20) -> bram0_20/3
  debus_addrb0/21(out20) -> bram0_20/4
  debus_dinb0/21(out20) -> bram0_20/5
  debus_web0/21(out20) -> bram0_20/6
  debus_addra0/22(out19) -> bram0_21/1
  debus_dina0/22(out19) -> bram0_21/2
  debus_wea0/22(out19) -> bram0_21/3
  debus_addrb0/22(out19) -> bram0_21/4
  debus_dinb0/22(out19) -> bram0_21/5
  debus_web0/22(out19) -> bram0_21/6
  debus_addra0/23(out18) -> bram0_22/1
  debus_dina0/23(out18) -> bram0_22/2
  debus_wea0/23(out18) -> bram0_22/3
  debus_addrb0/23(out18) -> bram0_22/4
  debus_dinb0/23(out18) -> bram0_22/5
  debus_web0/23(out18) -> bram0_22/6
  debus_addra0/24(out17) -> bram0_23/1
  debus_dina0/24(out17) -> bram0_23/2
  debus_wea0/24(out17) -> bram0_23/3
  debus_addrb0/24(out17) -> bram0_23/4
  debus_dinb0/24(out17) -> bram0_23/5
  debus_web0/24(out17) -> bram0_23/6
  debus_addra0/25(out16) -> bram0_24/1
  debus_dina0/25(out16) -> bram0_24/2
  debus_wea0/25(out16) -> bram0_24/3
  debus_addrb0/25(out16) -> bram0_24/4
  debus_dinb0/25(out16) -> bram0_24/5
  debus_web0/25(out16) -> bram0_24/6
  debus_addra0/26(out15) -> bram0_25/1
  debus_dina0/26(out15) -> bram0_25/2
  debus_wea0/26(out15) -> bram0_25/3
  debus_addrb0/26(out15) -> bram0_25/4
  debus_dinb0/26(out15) -> bram0_25/5
  debus_web0/26(out15) -> bram0_25/6
  debus_addra0/27(out14) -> bram0_26/1
  debus_dina0/27(out14) -> bram0_26/2
  debus_wea0/27(out14) -> bram0_26/3
  debus_addrb0/27(out14) -> bram0_26/4
  debus_dinb0/27(out14) -> bram0_26/5
  debus_web0/27(out14) -> bram0_26/6
  debus_addra0/28(out13) -> bram0_27/1
  debus_dina0/28(out13) -> bram0_27/2
  debus_wea0/28(out13) -> bram0_27/3
  debus_addrb0/28(out13) -> bram0_27/4
  debus_dinb0/28(out13) -> bram0_27/5
  debus_web0/28(out13) -> bram0_27/6
  debus_addra0/29(out12) -> bram0_28/1
  debus_dina0/29(out12) -> bram0_28/2
  debus_wea0/29(out12) -> bram0_28/3
  debus_addrb0/29(out12) -> bram0_28/4
  debus_dinb0/29(out12) -> bram0_28/5
  debus_web0/29(out12) -> bram0_28/6
  debus_addra0/30(out11) -> bram0_29/1
  debus_dina0/30(out11) -> bram0_29/2
  debus_wea0/30(out11) -> bram0_29/3
  debus_addrb0/30(out11) -> bram0_29/4
  debus_dinb0/30(out11) -> bram0_29/5
  debus_web0/30(out11) -> bram0_29/6
  debus_addra0/31(out10) -> bram0_30/1
  debus_dina0/31(out10) -> bram0_30/2
  debus_wea0/31(out10) -> bram0_30/3
  debus_addrb0/31(out10) -> bram0_30/4
  debus_dinb0/31(out10) -> bram0_30/5
  debus_web0/31(out10) -> bram0_30/6
  debus_addra0/32(out9) -> bram0_31/1
  debus_dina0/32(out9) -> bram0_31/2
  debus_wea0/32(out9) -> bram0_31/3
  debus_addrb0/32(out9) -> bram0_31/4
  debus_dinb0/32(out9) -> bram0_31/5
  debus_web0/32(out9) -> bram0_31/6
  debus_addra0/33(out8) -> bram0_32/1
  debus_dina0/33(out8) -> bram0_32/2
  debus_wea0/33(out8) -> bram0_32/3
  debus_addrb0/33(out8) -> bram0_32/4
  debus_dinb0/33(out8) -> bram0_32/5
  debus_web0/33(out8) -> bram0_32/6
  debus_addra0/34(out7) -> bram0_33/1
  debus_dina0/34(out7) -> bram0_33/2
  debus_wea0/34(out7) -> bram0_33/3
  debus_addrb0/34(out7) -> bram0_33/4
  debus_dinb0/34(out7) -> bram0_33/5
  debus_web0/34(out7) -> bram0_33/6
  debus_addra0/35(out6) -> bram0_34/1
  debus_dina0/35(out6) -> bram0_34/2
  debus_wea0/35(out6) -> bram0_34/3
  debus_addrb0/35(out6) -> bram0_34/4
  debus_dinb0/35(out6) -> bram0_34/5
  debus_web0/35(out6) -> bram0_34/6
  debus_addra0/36(out5) -> bram0_35/1
  debus_dina0/36(out5) -> bram0_35/2
  debus_wea0/36(out5) -> bram0_35/3
  debus_addrb0/36(out5) -> bram0_35/4
  debus_dinb0/36(out5) -> bram0_35/5
  debus_web0/36(out5) -> bram0_35/6
  debus_addra0/37(out4) -> bram0_36/1
  debus_dina0/37(out4) -> bram0_36/2
  debus_wea0/37(out4) -> bram0_36/3
  debus_addrb0/37(out4) -> bram0_36/4
  debus_dinb0/37(out4) -> bram0_36/5
  debus_web0/37(out4) -> bram0_36/6
  debus_addra0/38(out3) -> bram0_37/1
  debus_dina0/38(out3) -> bram0_37/2
  debus_wea0/38(out3) -> bram0_37/3
  debus_addrb0/38(out3) -> bram0_37/4
  debus_dinb0/38(out3) -> bram0_37/5
  debus_web0/38(out3) -> bram0_37/6
  debus_addra0/39(out2) -> bram0_38/1
  debus_dina0/39(out2) -> bram0_38/2
  debus_wea0/39(out2) -> bram0_38/3
  debus_addrb0/39(out2) -> bram0_38/4
  debus_dinb0/39(out2) -> bram0_38/5
  debus_web0/39(out2) -> bram0_38/6
  debus_addra0/40(lsb_out1) -> bram0_39/1
  debus_dina0/40(lsb_out1) -> bram0_39/2
  debus_wea0/40(lsb_out1) -> bram0_39/3
  debus_addrb0/40(lsb_out1) -> bram0_39/4
  debus_dinb0/40(lsb_out1) -> bram0_39/5
  debus_web0/40(lsb_out1) -> bram0_39/6
  bram0_0/1 -> A_bussify0/1(in1)
  bram0_0/2 -> B_bussify0/1(in1)
  bram0_1/1 -> A_bussify0/2(in2)
  bram0_1/2 -> B_bussify0/2(in2)
  bram0_2/1 -> A_bussify0/3(in3)
  bram0_2/2 -> B_bussify0/3(in3)
  bram0_3/1 -> A_bussify0/4(in4)
  bram0_3/2 -> B_bussify0/4(in4)
  bram0_4/1 -> A_bussify0/5(in5)
  bram0_4/2 -> B_bussify0/5(in5)
  bram0_5/1 -> A_bussify0/6(in6)
  bram0_5/2 -> B_bussify0/6(in6)
  bram0_6/1 -> A_bussify0/7(in7)
  bram0_6/2 -> B_bussify0/7(in7)
  bram0_7/1 -> A_bussify0/8(in8)
  bram0_7/2 -> B_bussify0/8(in8)
  bram0_8/1 -> A_bussify0/9(in9)
  bram0_8/2 -> B_bussify0/9(in9)
  bram0_9/1 -> A_bussify0/10(in10)
  bram0_9/2 -> B_bussify0/10(in10)
  bram0_10/1 -> A_bussify0/11(in11)
  bram0_10/2 -> B_bussify0/11(in11)
  bram0_11/1 -> A_bussify0/12(in12)
  bram0_11/2 -> B_bussify0/12(in12)
  bram0_12/1 -> A_bussify0/13(in13)
  bram0_12/2 -> B_bussify0/13(in13)
  bram0_13/1 -> A_bussify0/14(in14)
  bram0_13/2 -> B_bussify0/14(in14)
  bram0_14/1 -> A_bussify0/15(in15)
  bram0_14/2 -> B_bussify0/15(in15)
  bram0_15/1 -> A_bussify0/16(in16)
  bram0_15/2 -> B_bussify0/16(in16)
  bram0_16/1 -> A_bussify0/17(in17)
  bram0_16/2 -> B_bussify0/17(in17)
  bram0_17/1 -> A_bussify0/18(in18)
  bram0_17/2 -> B_bussify0/18(in18)
  bram0_18/1 -> A_bussify0/19(in19)
  bram0_18/2 -> B_bussify0/19(in19)
  bram0_19/1 -> A_bussify0/20(in20)
  bram0_19/2 -> B_bussify0/20(in20)
  bram0_20/1 -> A_bussify0/21(in21)
  bram0_20/2 -> B_bussify0/21(in21)
  bram0_21/1 -> A_bussify0/22(in22)
  bram0_21/2 -> B_bussify0/22(in22)
  bram0_22/1 -> A_bussify0/23(in23)
  bram0_22/2 -> B_bussify0/23(in23)
  bram0_23/1 -> A_bussify0/24(in24)
  bram0_23/2 -> B_bussify0/24(in24)
  bram0_24/1 -> A_bussify0/25(in25)
  bram0_24/2 -> B_bussify0/25(in25)
  bram0_25/1 -> A_bussify0/26(in26)
  bram0_25/2 -> B_bussify0/26(in26)
  bram0_26/1 -> A_bussify0/27(in27)
  bram0_26/2 -> B_bussify0/27(in27)
  bram0_27/1 -> A_bussify0/28(in28)
  bram0_27/2 -> B_bussify0/28(in28)
  bram0_28/1 -> A_bussify0/29(in29)
  bram0_28/2 -> B_bussify0/29(in29)
  bram0_29/1 -> A_bussify0/30(in30)
  bram0_29/2 -> B_bussify0/30(in30)
  bram0_30/1 -> A_bussify0/31(in31)
  bram0_30/2 -> B_bussify0/31(in31)
  bram0_31/1 -> A_bussify0/32(in32)
  bram0_31/2 -> B_bussify0/32(in32)
  bram0_32/1 -> A_bussify0/33(in33)
  bram0_32/2 -> B_bussify0/33(in33)
  bram0_33/1 -> A_bussify0/34(in34)
  bram0_33/2 -> B_bussify0/34(in34)
  bram0_34/1 -> A_bussify0/35(in35)
  bram0_34/2 -> B_bussify0/35(in35)
  bram0_35/1 -> A_bussify0/36(in36)
  bram0_35/2 -> B_bussify0/36(in36)
  bram0_36/1 -> A_bussify0/37(in37)
  bram0_36/2 -> B_bussify0/37(in37)
  bram0_37/1 -> A_bussify0/38(in38)
  bram0_37/2 -> B_bussify0/38(in38)
  bram0_38/1 -> A_bussify0/39(in39)
  bram0_38/2 -> B_bussify0/39(in39)
  bram0_39/1 -> A_bussify0/40(in40)
  bram0_39/2 -> B_bussify0/40(in40)
  A_bussify0/1(bus_out) -> A/1
  B_bussify0/1(bus_out) -> B/1

== system mymodel1/pfb_fir_generic/pfb_fir_taps/tap_split ==
  bus_in : Inport
  reinterpret{1..12} (12 alike) : xbsIndex_r4/Reinterpret  force_arith_type=on  arith_type=Unsigned  force_bin_pt=on  bin_pt=0  block_type=reinterpret
  slice1 : xbsIndex_r4/Slice  nbits=272  boolean_output=off  mode=Upper Bit Location + Width  bit1=-2992  base1=MSB of Input  bit0=0  base0=LSB of Input  dbl_ovrd=off  block_type=slice
  slice10 : xbsIndex_r4/Slice  nbits=272  boolean_output=off  mode=Upper Bit Location + Width  bit1=-544  base1=MSB of Input  bit0=0  base0=LSB of Input  dbl_ovrd=off  block_type=slice
  slice11 : xbsIndex_r4/Slice  nbits=272  boolean_output=off  mode=Upper Bit Location + Width  bit1=-272  base1=MSB of Input  bit0=0  base0=LSB of Input  dbl_ovrd=off  block_type=slice
  slice12 : xbsIndex_r4/Slice  nbits=272  boolean_output=off  mode=Upper Bit Location + Width  bit1=0  base1=MSB of Input  bit0=0  base0=LSB of Input  dbl_ovrd=off  block_type=slice
  slice2 : xbsIndex_r4/Slice  nbits=272  boolean_output=off  mode=Upper Bit Location + Width  bit1=-2720  base1=MSB of Input  bit0=0  base0=LSB of Input  dbl_ovrd=off  block_type=slice
  slice3 : xbsIndex_r4/Slice  nbits=272  boolean_output=off  mode=Upper Bit Location + Width  bit1=-2448  base1=MSB of Input  bit0=0  base0=LSB of Input  dbl_ovrd=off  block_type=slice
  slice4 : xbsIndex_r4/Slice  nbits=272  boolean_output=off  mode=Upper Bit Location + Width  bit1=-2176  base1=MSB of Input  bit0=0  base0=LSB of Input  dbl_ovrd=off  block_type=slice
  slice5 : xbsIndex_r4/Slice  nbits=272  boolean_output=off  mode=Upper Bit Location + Width  bit1=-1904  base1=MSB of Input  bit0=0  base0=LSB of Input  dbl_ovrd=off  block_type=slice
  slice6 : xbsIndex_r4/Slice  nbits=272  boolean_output=off  mode=Upper Bit Location + Width  bit1=-1632  base1=MSB of Input  bit0=0  base0=LSB of Input  dbl_ovrd=off  block_type=slice
  slice7 : xbsIndex_r4/Slice  nbits=272  boolean_output=off  mode=Upper Bit Location + Width  bit1=-1360  base1=MSB of Input  bit0=0  base0=LSB of Input  dbl_ovrd=off  block_type=slice
  slice8 : xbsIndex_r4/Slice  nbits=272  boolean_output=off  mode=Upper Bit Location + Width  bit1=-1088  base1=MSB of Input  bit0=0  base0=LSB of Input  dbl_ovrd=off  block_type=slice
  slice9 : xbsIndex_r4/Slice  nbits=272  boolean_output=off  mode=Upper Bit Location + Width  bit1=-816  base1=MSB of Input  bit0=0  base0=LSB of Input  dbl_ovrd=off  block_type=slice
  msb_out12 : Outport
  out11 : Outport  Port=2
  out10 : Outport  Port=3
  out9 : Outport  Port=4
  out8 : Outport  Port=5
  out7 : Outport  Port=6
  out6 : Outport  Port=7
  out5 : Outport  Port=8
  out4 : Outport  Port=9
  out3 : Outport  Port=10
  out2 : Outport  Port=11
  lsb_out1 : Outport  Port=12
  wires:
  bus_in/1 -> slice12/1, slice11/1, slice10/1, slice9/1, slice8/1, slice7/1, slice6/1, slice5/1, slice4/1, slice3/1, slice2/1, slice1/1
  slice12/1 -> reinterpret12/1
  reinterpret12/1 -> msb_out12/1
  slice11/1 -> reinterpret11/1
  reinterpret11/1 -> out11/1
  slice10/1 -> reinterpret10/1
  reinterpret10/1 -> out10/1
  slice9/1 -> reinterpret9/1
  reinterpret9/1 -> out9/1
  slice8/1 -> reinterpret8/1
  reinterpret8/1 -> out8/1
  slice7/1 -> reinterpret7/1
  reinterpret7/1 -> out7/1
  slice6/1 -> reinterpret6/1
  reinterpret6/1 -> out6/1
  slice5/1 -> reinterpret5/1
  reinterpret5/1 -> out5/1
  slice4/1 -> reinterpret4/1
  reinterpret4/1 -> out4/1
  slice3/1 -> reinterpret3/1
  reinterpret3/1 -> out3/1
  slice2/1 -> reinterpret2/1
  reinterpret2/1 -> out2/1
  slice1/1 -> reinterpret1/1
  reinterpret1/1 -> lsb_out1/1

== system mymodel1/simple_bram_vacc1/pulse_ext/posedge ==
  In : Inport
  Delay : xbsIndex_r4/Delay  rst=off  infoeditControl=Selection of Reset will increase slice count due to use of real FFs and instead of SRLs  en=off  latency=1  reg_retiming=off  dbl_ovrd=off  block_type=delay
      settings: xl_area=[0, 0, 0, 0, 0, 0, 0]
  Inverter : xbsIndex_r4/Inverter  en=off  latency=0  dbl_ovrd=off  block_type=inv
      settings: xl_area=[0, 0, 0, 0, 0, 0, 0]
  Logical : xbsIndex_r4/Logical  logical_function=AND  inputs=2  en=off  latency=0  precision=Full  arith_type=Unsigned  n_bits=8  bin_pt=2  align_bp=on  dbl_ovrd=off  block_type=logical
      settings: xl_area=[0, 0, 0, 0, 0, 0, 0]
  Out : Outport
  wires:
  Delay/1 -> Inverter/1
  Inverter/1 -> Logical/1
  In/1 -> Delay/1, Logical/2
  Logical/1 -> Out/1

== system mymodel1/simple_bram_vacc5/pulse_ext/posedge ==
  In : Inport
  Delay : xbsIndex_r4/Delay  rst=off  infoeditControl=Selection of Reset will increase slice count due to use of real FFs and instead of SRLs  en=off  latency=1  reg_retiming=off  dbl_ovrd=off  block_type=delay
      settings: xl_area=[0, 0, 0, 0, 0, 0, 0]
  Inverter : xbsIndex_r4/Inverter  en=off  latency=0  dbl_ovrd=off  block_type=inv
      settings: xl_area=[0, 0, 0, 0, 0, 0, 0]
  Logical : xbsIndex_r4/Logical  logical_function=AND  inputs=2  en=off  latency=0  precision=Full  arith_type=Unsigned  n_bits=8  bin_pt=2  align_bp=on  dbl_ovrd=off  block_type=logical
      settings: xl_area=[0, 0, 0, 0, 0, 0, 0]
  Out : Outport
  wires:
  Delay/1 -> Inverter/1
  Inverter/1 -> Logical/1
  In/1 -> Delay/1, Logical/2
  Logical/1 -> Out/1
